simulink model "chap4_9sim"  (Simulink 5.0)
settings: Solver=ode45  StartTime=0.0  StopTime=10  RelTol=1e-1
settings Model: LastModifiedBy=Administrator  ExtModeTrigMode=oneshot  ExtModeArmWhenConnect=off  LimitDataPoints=off  BooleanDataType=off

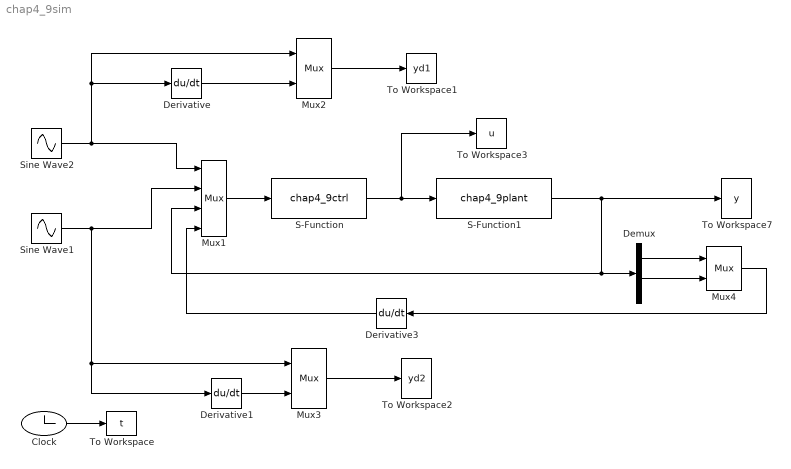
== system chap4_9sim ==
  Clock : Clock
  Demux : Demux  Outputs=6
  Derivative : Derivative
  Derivative1 : Derivative
  Derivative3 : Derivative  Orientation=left
  Mux1 : Mux
  Mux2 : Mux  Inputs=2
  Mux3 : Mux  Inputs=2
  Mux4 : Mux  Inputs=2
  S-Function : S-Function  FunctionName=chap4_9ctrl
  S-Function1 : S-Function  FunctionName=chap4_9plant
  Sine Wave1 : Sin  Amplitude=0.3  SampleTime=0
  Sine Wave2 : Sin  Amplitude=0.3  SampleTime=0
  To Workspace : ToWorkspace  VariableName=t  SampleTime=-1  SaveFormat=Array
  To Workspace1 : ToWorkspace  VariableName=yd1  SampleTime=-1  SaveFormat=Array
  To Workspace2 : ToWorkspace  VariableName=yd2  SampleTime=-1  SaveFormat=Array
  To Workspace3 : ToWorkspace  VariableName=u  SampleTime=-1  SaveFormat=Array
  To Workspace7 : ToWorkspace  VariableName=y  SampleTime=-1  SaveFormat=Array
  wires:
  Clock/1 -> To Workspace/1
  S-Function/1 -> S-Function1/1, To Workspace3/1
  Sine Wave2/1 -> Mux1/1, Derivative/1, Mux2/1
  Sine Wave1/1 -> Mux1/2, Derivative1/1, Mux3/1
  S-Function1/1 -> To Workspace7/1, Mux1/3, Demux/1
  Mux1/1 -> S-Function/1
  Mux2/1 -> To Workspace1/1
  Derivative/1 -> Mux2/2
  Mux3/1 -> To Workspace2/1
  Derivative1/1 -> Mux3/2
  Derivative3/1 -> Mux1/4
  Demux/2 -> Mux4/1
  Demux/4 -> Mux4/2
  Mux4/1 -> Derivative3/1
